simulink model "Pure_Pursuit"  (R2025b)
settings: Solver=FixedStepAuto  StartTime=0.0  StopTime=98.5383  FixedStep=0.01  RelTol=1e-3  EnableMultiTasking=on
values from neighbouring files (symbols this model uses):
  L = 0.2    [untitled2.m]
  P = densifyPath(path, 0.05)    [untitled2.m]
  start = [1 1]    [untitled2.m]
  theta0 = atan2(P(2,2) - P(1,2), P(2,1) - P(1,1))    [untitled2.m]
libraries: slpidlib x2, robotalgslib x1
settings Model: Creator=mwali  LastModifiedBy=mwali
settings OptimizationCC: DefaultParameterBehavior=Inlined  EnhancedBackFolding=on  PassReuseOutputArgsAs=Individual arguments  ZeroExternalMemoryAtStartup=off  ZeroInternalMemoryAtStartup=off  MaxStackSize=64  OptimizeBlockOrder=speed  DifferentSizesBufferReuse=on  EfficientTunableParamExpr=on
settings DebuggingCC: ParameterTunabilityLossMsg=error
settings HardwareCC: ProdBitPerPointer=32.0  ProdBitPerSizeT=32.0  ProdBitPerPtrDiffT=32.0  ProdLargestAtomicInteger=Long  ProdLargestAtomicFloat=Double  ProdWordSize=32.0  ProdLongLongMode=on  ProdHWDeviceType=ARM Compatible->ARM Cortex-M
settings SFSimCC: MATLABDynamicMemAlloc=off
settings RTWCC: SystemTargetFile=ert.tlc  GenCodeOnly=on  TemplateMakefile=ert_default_tmf  Description=Embedded Coder
settings CodeAppCC: ForceParamTrailComments=on  IgnoreCustomStorageClasses=off  OperatorAnnotations=on  SimulinkDataObjDesc=on  SFDataObjDesc=on  InsertBlockDesc=on
settings ERTTargetCC: ExtModeTransport=3.0  ExtModeStaticAlloc=on  ExtModeStaticAllocSize=2048.0  ExtModeMexFile=ext_xcp  ExtModeIntrfLevel=Level2 - Open  ERTCustomFileTemplate=example_file_process.tlc  TargetLangStandard=C99 (ISO)  CodeReplacementLibrary=ARM Cortex-M

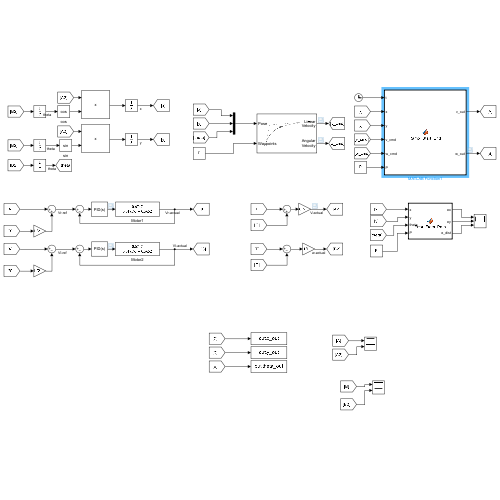
[thumbnail: Simulink's stored preview of the top-level diagram]
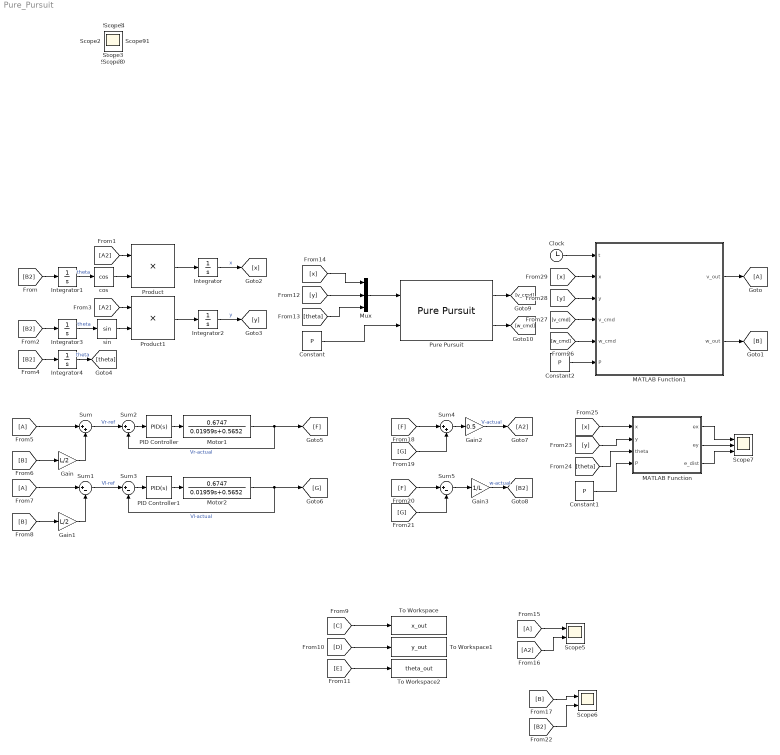
== system Pure_Pursuit ==
  Clock : Clock
  Constant : Constant  Value=P
  Constant1 : Constant  Value=P
  Constant2 : Constant  Value=P
  From15 : From
  From5 : From
  From7 : From
  Gain : Gain  Gain=L/2
  Gain1 : Gain  Gain=L/2
  Gain2 : Gain  Gain=0.5
  Gain3 : Gain  Gain=1/L
  Goto : Goto
  Integrator : Integrator  InitialCondition=start(1)
  Integrator1 : Integrator  InitialCondition=theta0
  Integrator2 : Integrator  InitialCondition=start(2)
  Integrator3 : Integrator  InitialCondition=theta0
  Integrator4 : Integrator  InitialCondition=theta0
  MATLAB Function : MATLAB Function  TreatAsAtomicUnit=on
  MATLAB Function1 : MATLAB Function  TreatAsAtomicUnit=on
  Motor1 : TransferFcn  Numerator=[0.6747]  Denominator=[0.01959 0.5652]
  Motor2 : TransferFcn  Numerator=[0.6747]  Denominator=[0.01959 0.5652]
  Mux : Mux  Inputs=3
  PID Controller : slpidlib/PID Controller  Controller=PID  Form=Parallel  TimeDomain=Continuous-time  UseExternalTs=off  SampleTime=-1  IntegratorMethod=Forward Euler  FilterMethod=Forward Euler  ControllerParametersSource=internal  P=1.12049858212093  I=0.5  UseKiTs=off  D=-0.00141040716856919  UseExternalDerivativeSource=off  N=109.085667259497  UseFilter=on  TunerSelectOption=Transfer Function Based (PID Tuner App)  InitialConditionSource=internal  InitialConditionForIntegrator=0  InitialConditionForFilter=0  DifferentiatorICPrevScaledInput=0  ExternalReset=none  TrackingMode=off  Kt=1  LimitOutput=off  SatLimitsSource=internal  UpperSaturationLimit=inf  LowerSaturationLimit=-inf  LinearizeAsGain=on  AntiWindupMode=none  Kb=1  LimitIntegrator=off  UpperIntegratorSaturationLimit=inf  LowerIntegratorSaturationLimit=-inf  POutMin=[]  POutMax=[]  IOutMin=[]  IOutMax=[]  DOutMin=[]  DOutMax=[]  NOutMin=[]  NOutMax=[]  SumOutMin=[]  SumOutMax=[]  SaturationOutMin=[]  SaturationOutMax=[]  PParamMin=[]  PParamMax=[]  IParamMin=[]  IParamMax=[]  DParamMin=[]  DParamMax=[]  NParamMin=[]  NParamMax=[]  KbParamMin=[]  KbParamMax=[]  KtParamMin=[]  KtParamMax=[]  KbOutMin=[]  KbOutMax=[]  KtOutMin=[]  KtOutMax=[]  IntegratorOutMin=[]  IntegratorOutMax=[]  FilterOutMin=[]  FilterOutMax=[]  SumI1OutMin=[]  SumI1OutMax=[]  SumI2OutMin=[]  SumI2OutMax=[]  SumI3OutMin=[]  SumI3OutMax=[]  SumI4OutMin=[]  SumI4OutMax=[]  SumDOutMin=[]  SumDOutMax=[]  DifferentiatorOutMin=[]  DifferentiatorOutMax=[]  FilterDiffOutCoefMin=[]  FilterDiffOutCoefMax=[]  ReciprocalOutMin=[]  ReciprocalOutMax=[]  SumDenOutMin=[]  SumDenOutMax=[]  SumNumOutMin=[]  SumNumOutMax=[]  DivideOutMin=[]  DivideOutMax=[]  UdiffTsProdOutMin=[]  UdiffTsProdOutMax=[]  NTsProdOutMin=[]  NTsProdOutMax=[]  UintegralTsProdOutMin=[]  UintegralTsProdOutMax=[]  UngainTsProdOutMin=[]  UngainTsProdOutMax=[]  ClampingZeroOutDataTypeStr=Inherit: Inherit via back propagation  ClampingZeroOutMin=[]  ClampingZeroOutMax=[]  FilterDenConstantOutDataTypeStr=Inherit: Inherit via back propagation  FilterDenConstantOutMin=[]  FilterDenConstantOutMax=[]  PCopyOutDataTypeStr=Inherit: Inherit via back propagation  PCopyOutMin=[]  PCopyOutMax=[]  NCopyOutDataTypeStr=Inherit: Inherit via back propagation  NCopyOutMin=[]  NCopyOutMax=[]  IntegratorContinuousStateAttributes=''  IntegratorStateMustResolveToSignalObject=off  IntegratorRTWStateStorageClass=Auto  FilterContinuousStateAttributes=''  FilterStateMustResolveToSignalObject=off  FilterRTWStateStorageClass=Auto  ParallelPVariant=InternalParameters  IdealPVariant=Disabled  IVariant=InternalParameters  DVariant=InternalParameters  IntegratorVariant=Continuous  SatVariant=Disabled  AWVariant=Passthrough  PCopyVariant=Disabled  TRVariant=Disabled  FdbkBlocksVariant=Forward  IdealPFdbkVariant=Disabled  SatFdbkVariant=Disabled  DerivativeFilterVariant=ContFilter  NVariant=InternalParameters  NCopyVariant=Disabled  FilterICVariant=InternalICsFilter  IntegratorICVariant=InternalICs  ExternalResetVariant=Disabled  TRSumVariant=Passthrough  SumFdbkVariant=Disabled  SumVariant=Sum_PID  TsampFilterVariant=InternalTs  TsampNgainVariant=Passthrough  TsampIntegralVariant=Disabled_SignalSpec  ExternalSaturationOutDataTypeStr=Inherit: Same as second input  DerivativeSourceVariant=ErrorSignal  PreIntVariant=InternalPreInt
  PID Controller1 : slpidlib/PID Controller  Controller=PID  Form=Parallel  TimeDomain=Continuous-time  UseExternalTs=off  SampleTime=-1  IntegratorMethod=Forward Euler  FilterMethod=Forward Euler  ControllerParametersSource=internal  P=1.12049858212093  I=0.5  UseKiTs=off  D=-0.00141040716856919  UseExternalDerivativeSource=off  N=109.085667259497  UseFilter=on  TunerSelectOption=Transfer Function Based (PID Tuner App)  InitialConditionSource=internal  InitialConditionForIntegrator=0  InitialConditionForFilter=0  DifferentiatorICPrevScaledInput=0  ExternalReset=none  TrackingMode=off  Kt=1  LimitOutput=off  SatLimitsSource=internal  UpperSaturationLimit=inf  LowerSaturationLimit=-inf  LinearizeAsGain=on  AntiWindupMode=none  Kb=1  LimitIntegrator=off  UpperIntegratorSaturationLimit=inf  LowerIntegratorSaturationLimit=-inf  POutMin=[]  POutMax=[]  IOutMin=[]  IOutMax=[]  DOutMin=[]  DOutMax=[]  NOutMin=[]  NOutMax=[]  SumOutMin=[]  SumOutMax=[]  SaturationOutMin=[]  SaturationOutMax=[]  PParamMin=[]  PParamMax=[]  IParamMin=[]  IParamMax=[]  DParamMin=[]  DParamMax=[]  NParamMin=[]  NParamMax=[]  KbParamMin=[]  KbParamMax=[]  KtParamMin=[]  KtParamMax=[]  KbOutMin=[]  KbOutMax=[]  KtOutMin=[]  KtOutMax=[]  IntegratorOutMin=[]  IntegratorOutMax=[]  FilterOutMin=[]  FilterOutMax=[]  SumI1OutMin=[]  SumI1OutMax=[]  SumI2OutMin=[]  SumI2OutMax=[]  SumI3OutMin=[]  SumI3OutMax=[]  SumI4OutMin=[]  SumI4OutMax=[]  SumDOutMin=[]  SumDOutMax=[]  DifferentiatorOutMin=[]  DifferentiatorOutMax=[]  FilterDiffOutCoefMin=[]  FilterDiffOutCoefMax=[]  ReciprocalOutMin=[]  ReciprocalOutMax=[]  SumDenOutMin=[]  SumDenOutMax=[]  SumNumOutMin=[]  SumNumOutMax=[]  DivideOutMin=[]  DivideOutMax=[]  UdiffTsProdOutMin=[]  UdiffTsProdOutMax=[]  NTsProdOutMin=[]  NTsProdOutMax=[]  UintegralTsProdOutMin=[]  UintegralTsProdOutMax=[]  UngainTsProdOutMin=[]  UngainTsProdOutMax=[]  ClampingZeroOutDataTypeStr=Inherit: Inherit via back propagation  ClampingZeroOutMin=[]  ClampingZeroOutMax=[]  FilterDenConstantOutDataTypeStr=Inherit: Inherit via back propagation  FilterDenConstantOutMin=[]  FilterDenConstantOutMax=[]  PCopyOutDataTypeStr=Inherit: Inherit via back propagation  PCopyOutMin=[]  PCopyOutMax=[]  NCopyOutDataTypeStr=Inherit: Inherit via back propagation  NCopyOutMin=[]  NCopyOutMax=[]  IntegratorContinuousStateAttributes=''  IntegratorStateMustResolveToSignalObject=off  IntegratorRTWStateStorageClass=Auto  FilterContinuousStateAttributes=''  FilterStateMustResolveToSignalObject=off  FilterRTWStateStorageClass=Auto  ParallelPVariant=InternalParameters  IdealPVariant=Disabled  IVariant=InternalParameters  DVariant=InternalParameters  IntegratorVariant=Continuous  SatVariant=Disabled  AWVariant=Passthrough  PCopyVariant=Disabled  TRVariant=Disabled  FdbkBlocksVariant=Forward  IdealPFdbkVariant=Disabled  SatFdbkVariant=Disabled  DerivativeFilterVariant=ContFilter  NVariant=InternalParameters  NCopyVariant=Disabled  FilterICVariant=InternalICsFilter  IntegratorICVariant=InternalICs  ExternalResetVariant=Disabled  TRSumVariant=Passthrough  SumFdbkVariant=Disabled  SumVariant=Sum_PID  TsampFilterVariant=InternalTs  TsampNgainVariant=Passthrough  TsampIntegralVariant=Disabled_SignalSpec  ExternalSaturationOutDataTypeStr=Inherit: Same as second input  DerivativeSourceVariant=ErrorSignal  PreIntVariant=InternalPreInt
  Product : Product
  Product1 : Product
  Pure Pursuit : robotalgslib/Pure Pursuit  DesiredLinearVelocityPort=off  DesiredLinearVelocity=0.15  MaxAngularVelocity=3  LookaheadDistancePort=off  LookaheadDistance=0.2  TargetDirPort=off  SimulateUsing=Interpreted execution
      settings: LibrarySourceBlock=robotmobilelib/Pure Pursuit
  Scope5 : Scope  NumInputPorts=2
      settings: ActiveDisplayYMinimum=-0.018750000000000006  ActiveDisplayYMaximum=0.16875000000000009  DataLoggingVariableName=ScopeData5
  Scope6 : Scope  NumInputPorts=2
      settings: ActiveDisplayYMinimum=-1  ActiveDisplayYMaximum=1  DataLoggingVariableName=ScopeData6
  Scope7 : Scope  NumInputPorts=3
      settings: ActiveDisplayYMinimum=-0.18805745911739136  ActiveDisplayYMaximum=0.29573072852786447  DataLoggingVariableName=ScopeData7
  Sum : Sum  Inputs=|++
  Sum{1..3,5} (4 alike) : Sum  Inputs=|+-
  Sum4 : Sum  Inputs=|++
  To Workspace : ToWorkspace  VariableName=x_out  SampleTime=-1
  To Workspace1 : ToWorkspace  VariableName=y_out  SampleTime=-1
  To Workspace2 : ToWorkspace  VariableName=theta_out  SampleTime=-1
  cos : Trigonometry  Operator=cos
  sin : Trigonometry
  Scope{,1..4,8..11} (9 alike) : Scope
      Scope settings: ActiveDisplayYMinimum=-0.037808986482854419  ActiveDisplayYMaximum=0.34028087834568982
      Scope1 settings: ActiveDisplayYMinimum=-1  ActiveDisplayYMaximum=1
      Scope10 settings: ActiveDisplayYMinimum=-0.62934086108777831  ActiveDisplayYMaximum=3.4032600956764196  DataLoggingVariableName=ScopeData10
      Scope11 settings: ActiveDisplayYMinimum=-0.018749999777632118  ActiveDisplayYMaximum=0.16874999799868909  DataLoggingVariableName=ScopeData11
      Scope2 settings: ActiveDisplayYMinimum=-1  ActiveDisplayYMaximum=1  DataLoggingVariableName=ScopeData2
      Scope3 settings: ActiveDisplayYMinimum=-1  ActiveDisplayYMaximum=1  DataLoggingVariableName=ScopeData3
      Scope4 settings: ActiveDisplayYMinimum=6.9294550712517484  ActiveDisplayYMaximum=7.321549507751806  DataLoggingVariableName=ScopeData4
      Scope8 settings: ActiveDisplayYMinimum=-0.041963530010024855  ActiveDisplayYMaximum=0.37767177009022374  DataLoggingVariableName=ScopeData8
      Scope9 settings: ActiveDisplayYMinimum=-1  ActiveDisplayYMaximum=1  DataLoggingVariableName=ScopeData9
  wires:
  Product/1 -> Integrator/1
  cos/1 -> Product/2
  Integrator1/1 -> cos/1  "theta"
  [B2] -> Integrator1/1
  [A2] -> Product/1
  sin/1 -> Product1/2
  [B2] -> Integrator3/1
  Product1/1 -> Integrator2/1
  [A2] -> Product1/1
  Integrator3/1 -> sin/1  "theta"
  [B2] -> Integrator4/1
  Mux/1 -> Pure Pursuit/1
  Constant/1 -> Pure Pursuit/2
  [B] -> Gain/1
  From5/1 -> Sum/1
  Gain/1 -> Sum/2
  From7/1 -> Sum1/1
  Gain1/1 -> Sum1/2
  [B] -> Gain1/1
  Integrator/1 -> [x]  "x"
  Integrator2/1 -> [y]  "y"
  Integrator4/1 -> [theta]  "theta"
  [C] -> To Workspace/1
  [D] -> To Workspace1/1
  [E] -> To Workspace2/1
  [x] -> Mux/1
  [y] -> Mux/2
  [theta] -> Mux/3
  Sum/1 -> Sum2/1  "Vr-ref"
  Sum2/1 -> PID Controller/1
  Motor1/1 -> [F], Sum2/2  "Vr-actual"
  Motor2/1 -> Sum3/2, [G]  "Vl-actual"
  Sum3/1 -> PID Controller1/1
  Sum1/1 -> Sum3/1  "Vl-ref"
  [F] -> Sum4/1
  [G] -> Sum4/2
  Sum4/1 -> Gain2/1
  Gain2/1 -> [A2]  "V-actual"
  [F] -> Sum5/1
  [G] -> Sum5/2
  Sum5/1 -> Gain3/1
  Gain3/1 -> [B2]  "w-actual"
  PID Controller/1 -> Motor1/1
  PID Controller1/1 -> Motor2/1
  From15/1 -> Scope5/1
  [A2] -> Scope5/2
  [B] -> Scope6/1
  [B2] -> Scope6/2
  [theta] -> MATLAB Function/3(theta)
  [x] -> MATLAB Function/1(x)
  [y] -> MATLAB Function/2(y)
  Constant1/1 -> MATLAB Function/4(P)
  MATLAB Function/1(ex) -> Scope7/1
  MATLAB Function/2(ey) -> Scope7/2
  MATLAB Function/3(e_dist) -> Scope7/3
  [x] -> MATLAB Function1/2(x)
  [y] -> MATLAB Function1/3(y)
  Constant2/1 -> MATLAB Function1/6(P)
  MATLAB Function1/1(v_out) -> Goto/1
  MATLAB Function1/2(w_out) -> [B]
  Clock/1 -> MATLAB Function1/1(t)
  Pure Pursuit/1 -> [v_cmd]
  Pure Pursuit/2 -> [w_cmd]
  [v_cmd] -> MATLAB Function1/4(v_cmd)
  [w_cmd] -> MATLAB Function1/5(w_cmd)

== matlab function Pure_Pursuit/MATLAB Function1 ==
  data: t input; x input; v_out output; y input; v_cmd input; w_cmd input; P input; w_out output
function [v_out, w_out] = Ramp_Start_End(t, x, y, v_cmd, w_cmd, P)

% Final goal = last waypoint
goalX = P(end,1);
goalY = P(end,2);

dx = goalX - x;
dy = goalY - y;
distToGoal = sqrt(dx^2 + dy^2);

% Settings
T_startRamp = 5.0;     % first 5 seconds ramp up
T_endRamp   = 5.0;     % last 5 seconds ramp down

v_nominal  = 0.12;     % put your normal speed here
stopRadius = 0.10;     % stop within 10 cm

% Distance needed for 5 seconds ramp down
rampDownDistance = v_nominal * T_endRamp;

% -------------------------
% Start ramp: 0 to 1
% -------------------------
startScale = t / T_startRamp;

if startScale > 1
    startScale = 1;
elseif startScale < 0
    startScale = 0;
end

% -------------------------
% End ramp: 1 to 0
% -------------------------
if distToGoal <= stopRadius
    endScale = 0;
elseif distToGoal <= rampDownDistance
    endScale = (distToGoal - stopRadius) / (rampDownDistance - stopRadius);
else
    endScale = 1;
end

if endScale > 1
    endScale = 1;
elseif endScale < 0
    endScale = 0;
end

% Final scale
scale = startScale * endScale;

% Apply ramp to Pure Pursuit commands
v_out = scale * v_cmd;
w_out = scale * w_cmd;

% Final stop
if distToGoal <= stopRadius
    atGoal = true;
    v_out = 0;
    w_out = 0;
else
    atGoal = false;
end

end

== matlab function Pure_Pursuit/MATLAB Function ==
  data: x input; ex output; y input; theta input; P input; ey output; e_dist output
function [ex, ey, e_dist] = Error_From_Path(x, y, theta, P)

% P is the path waypoints
% P(:,1) = x path points
% P(:,2) = y path points

N = size(P,1);

minDist = inf;
nearestIndex = 1;

% Find nearest point on the path
for i = 1:N
    dx_i = P(i,1) - x;
    dy_i = P(i,2) - y;
    dist_i = dx_i^2 + dy_i^2;

    if dist_i < minDist
        minDist = dist_i;
        nearestIndex = i;
    end
end

% Internal desired point only
xd = P(nearestIndex,1);
yd = P(nearestIndex,2);

% Error between robot and nearest path point
dx = xd - x;
dy = yd - y;

% Error in robot frame
ex = cos(theta)*dx + sin(theta)*dy;
ey = -sin(theta)*dx + cos(theta)*dy;

% Absolute distance error
e_dist = sqrt(dx^2 + dy^2);

end
